simulink model "Quad_Observer_Psi"  (Simulink 7.7)
settings: Solver=ode45  StartTime=0.0  StopTime=1  RelTol=1e-3
undefined symbols (not defined in the file or in its folder): quad
settings Model: Creator=Alexey  LastModifiedBy=Alexey

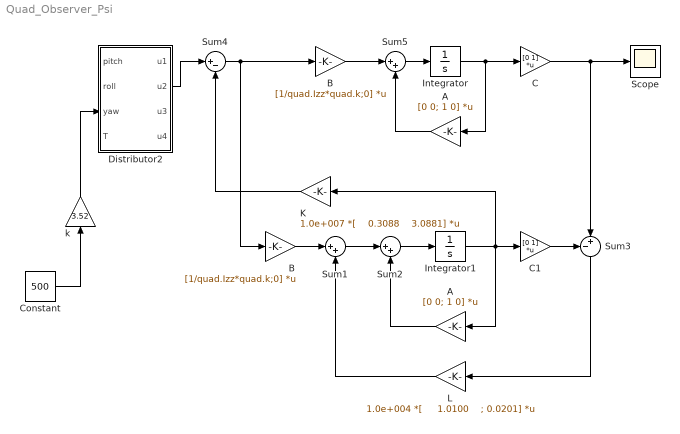
== system Quad_Observer_Psi ==
  A : Gain  Gain=[0 0; 1 0]  Multiplication=Matrix(K*u)
  "A " : Gain  Gain=[0 0; 1 0]  Multiplication=Matrix(K*u)
  B : Gain  Gain=[1/quad.Izz*quad.k;0]  Multiplication=Matrix(K*u)
  "B " : Gain  Gain=[1/quad.Izz*quad.k;0]  Multiplication=Matrix(K*u)
  C : Gain  Gain=[0 1]  Multiplication=Matrix(K*u)
  C1 : Gain  Gain=[0 1]  Multiplication=Matrix(K*u)
  Constant : Constant  Value=500
  Distributor2 : Subsystem
  Integrator : Integrator
  Integrator1 : Integrator
  K : Gain  Gain="1.0e+007 *[    0.3088    3.0881]"  Multiplication=Matrix(K*u)
  L : Gain  Gain=|  Multiplication=Matrix(K*u)
      | 1.0e+004 *[
      | 
      |     1.0100
      |    ; 0.0201]
  Scope : Scope
  Sum1 : Sum  Inputs=|++
  Sum2 : Sum  Inputs=|++
  Sum3 : Sum  Inputs=-+|
  Sum4 : Sum  Inputs=|+-
  Sum5 : Sum  Inputs=|++
  k : Gain  Gain=3.52
  wires:
  Sum4/1 -> B/1, "B "/1
  B/1 -> Sum5/1
  Sum5/1 -> Integrator/1
  Integrator/1 -> C/1, "A "/1
  C/1 -> Sum3/2, Scope/1
  "A "/1 -> Sum5/2
  Sum1/1 -> Sum2/1
  Sum2/1 -> Integrator1/1
  Integrator1/1 -> K/1, C1/1, A/1
  C1/1 -> Sum3/1
  A/1 -> Sum2/2
  Sum3/1 -> L/1
  L/1 -> Sum1/2
  K/1 -> Sum4/2
  "B "/1 -> Sum1/1
  Constant/1 -> k/1
  k/1 -> Distributor2/3(yaw)
  Distributor2/2("u2 ") -> Sum4/1

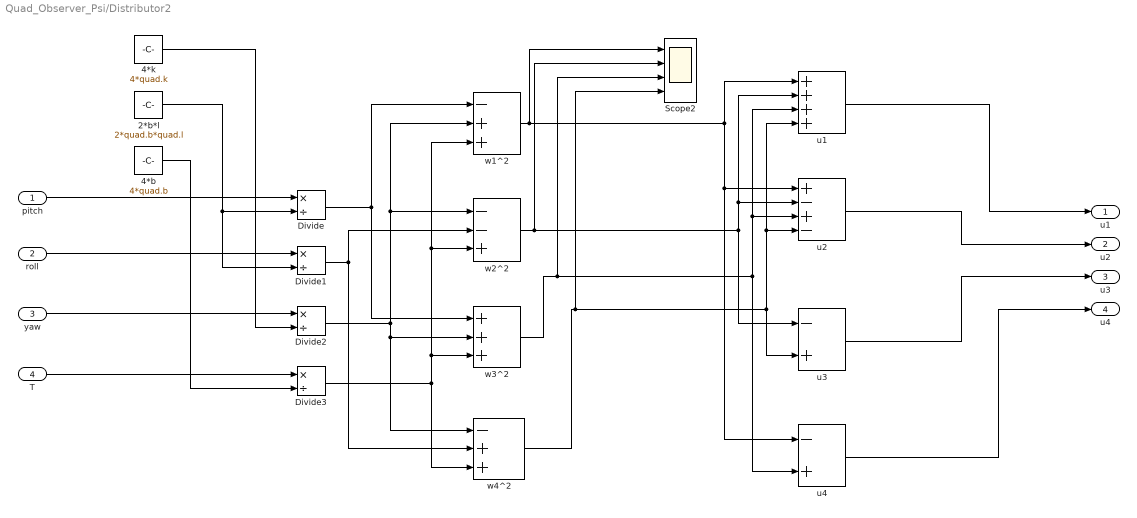
== system Quad_Observer_Psi/Distributor2 ==
  pitch : Inport
  roll : Inport  Port=2
  yaw : Inport  Port=3
  T : Inport  Port=4
  2*b*l : Constant  Value=2*quad.b*quad.l
  4*b : Constant  Value=4*quad.b
  4*k : Constant  Value=4*quad.k
  Divide{,1..3} (4 alike) : Product  Inputs=*/
  Scope2 : Scope  NumInputPorts=4
      settings: YMin=-1.5e+007~-2.5e+006~-1.5e+007~-2.5e+006  YMax=2.5e+006~1.25e+007~2.5e+006~1.25e+007  SaveName=ScopeData9
  u1 : Sum  Inputs=++++
  u2 : Sum  Inputs=+-+-
  u3 : Sum  Inputs=-+
  u4 : Sum  Inputs=-+
  w1^2 : Sum  Inputs=-++
  w2^2 : Sum  Inputs=--+
  w3^2 : Sum  Inputs=+++
  w4^2 : Sum  Inputs=-++
  "u1 " : Outport
  "u2 " : Outport  Port=2
  "u3 " : Outport  Port=3
  "u4 " : Outport  Port=4
  wires:
  4*k/1 -> Divide2/2
  Divide1/1 -> w4^2/2, w2^2/2
  Divide2/1 -> w3^2/2, w4^2/1, w2^2/1, w1^2/2
  Divide/1 -> w3^2/1, w1^2/1
  4*b/1 -> Divide3/2
  yaw/1 -> Divide2/1
  2*b*l/1 -> Divide/2, Divide1/2
  roll/1 -> Divide1/1
  pitch/1 -> Divide/1
  w1^2/1 -> Scope2/1, u1/1, u2/1, u4/1
  w2^2/1 -> Scope2/2, u1/2, u2/2, u3/1
  w3^2/1 -> Scope2/3, u1/3, u2/3, u4/2
  w4^2/1 -> Scope2/4, u1/4, u2/4, u3/2
  Divide3/1 -> w2^2/3, w1^2/3, w3^2/3, w4^2/3
  T/1 -> Divide3/1
  u1/1 -> "u1 "/1
  u2/1 -> "u2 "/1
  u3/1 -> "u3 "/1
  u4/1 -> "u4 "/1
